simulink model "Sim_model"  (R2024a)
settings: Solver=ode23t  StartTime=0.0  StopTime=7  FixedStep=0.01  MaxStep=0.05  RelTol=1e-3  EnableMultiTasking=on
PreLoadFcn:
  | mdl_puma560
undefined symbols (not defined in the file or in its folder): p560, slcoulomb
libraries: roblocks x3
settings Model: Creator=pic  LastModifiedBy=nicolasaltarelli
settings SolverCC: ZeroCrossControl=DisableAll  AlgebraicLoopSolver=TrustRegion
settings DataIOCC: SaveFormat=Array  SignalLoggingSaveFormat=ModelDataLogs  ReturnWorkspaceOutputs=off  TimeSaveName=t  OutputSaveName=y  ReturnWorkspaceOutputsName=ctorque
settings OptimizationCC: BlockReduction=off  BooleanDataType=off  ExpressionDepthLimit=2147483647  InitFltsAndDblsToZero=on  LifeSpan=inf
settings DebuggingCC: SaveWithParameterizedLinksMsg=none  UnderspecifiedInitializationDetection=Classic  MergeDetectMultiDrivingBlocksExec=none  SignalResolutionControl=TryResolveAllWithWarning  MultiTaskDSMMsg=warning  MultiTaskCondExecSysMsg=none  FcnCallInpInsideContextMsg=warning  UnconnectedInputMsg=warning  UnconnectedOutputMsg=warning  UnconnectedLineMsg=warning  AllowSymbolicDim=off  StateNameClashWarn=warning  SFUnexpectedBacktrackingDiag=warning  SFNoUnconditionalDefaultTransitionDiag=warning  SFExecutionAtInitializationDiag=none  ArithmeticOperatorsInVariantConditions=warning
settings HardwareCC: ProdBitPerPointer=32  ProdBitPerSizeT=32  ProdBitPerPtrDiffT=32  ProdLargestAtomicFloat=None  ProdIntDivRoundTo=Undefined  ProdEndianess=Unspecified  ProdWordSize=32  ProdHWDeviceType=32-bit Generic  TargetUnknown=on
settings ModelReferenceCC: EnableRefExpFcnMdlSchedulingChecks=on  PropagateSignalLabelsOutOfModel=off
settings SFSimCC: SimUseLocalCustomCode=off  CustomCodeUndefinedFunction=UseInterfaceOnly
settings RTWCC: RTWUseLocalCustomCode=off  GPUComputeCapability=3.5
settings CodeAppCC: StateflowObjectComments=on
settings GRTTargetCC: TargetLangStandard=C89/C90 (ANSI)  ModelReferenceCompliant=off  CompOptLevelCompliant=off  CombineOutputUpdateFcns=off  MatFileLogging=off  GRTInterface=on
settings ConfigComp: CovMetricSettings=dw  CovSaveCumulativeToWorkspaceVar=on  CovSaveSingleToWorkspaceVar=on  CovExternalEMLEnable=off

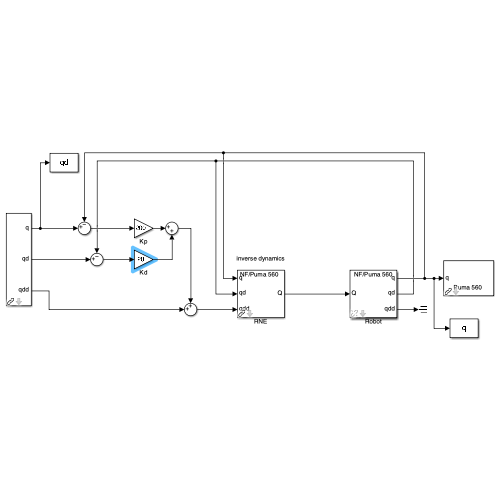
[thumbnail: Simulink's stored preview of the top-level diagram]
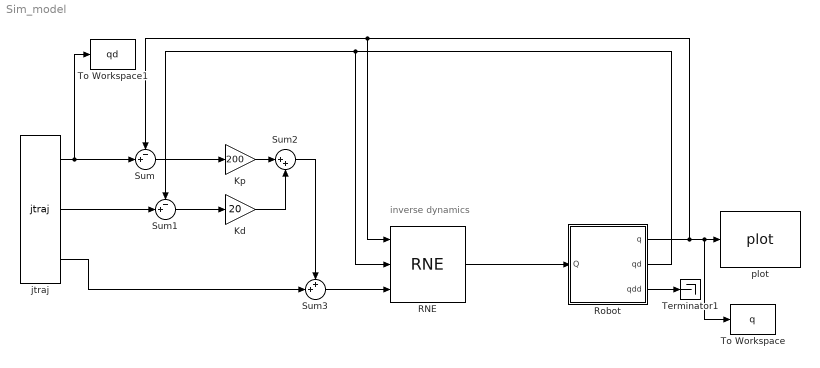
== system Sim_model ==
  note: inverse dynamics
  Kd : Gain  Gain=20  SaturateOnIntegerOverflow=on  OutDataTypeStr=Inherit: Same as input  ParamDataTypeStr=Inherit: Same as input
  Kp : Gain  Gain=200  SaturateOnIntegerOverflow=on  OutDataTypeStr=Inherit: Same as input  ParamDataTypeStr=Inherit: Same as input
  RNE : roblocks/Arm/RNE  robot=p2.nofriction  grav=[0 0 9.81]
  Robot : Subsystem  AncestorBlock=roblocks/Arm/Robot  mask{robot=p560.nofriction, q0=[0 0 0 0 0 0]}
      mask prompts: robot "Robot object"; q0 "Initial state"
      mask help: Rigid-body dynamic model of robot.
      mask init:
      | if isa(robot, 'SerialLink')
      |     rname = robot.name;
      |     %fprintf('**robot name is %s\n', rname);
      | else
      |     rname = '';
      |     n = 0
      | end
      mask Help:
      | Simulates the forward (direct) rigid-body dynamics of the robot described
      | by the given robot object.  For given applied joint torque/force it computes
      | the instaneous joint coordinates, velocities and acclerations.
      | 
      | 
      | <b>Parameters::</b>
      | 
      | robot (SerialLink) a dynamic model of an N-link serial link manipulator
      | q0 (1xN)  Initial joint coordinates
      | 
      | <b>Inputs::</b>
      | 
      | Q (1xN) the generalized joint force (torque or force) required to achieve
      | the motion state (q, qd, qdd).
      | 
      | <b>Outputs::</b>
      | 
      | q (1xN) joint coordinates
      | qd (1xN) joint coordinate velocity
      | qdd (1xN) joint coordinate acceleration
      | 
      | 
      | <b>Notes::</b>
      | 
      | - Required to simulate robot rigid body motion.
      | - Implemented using the recursive Newton-Euler scheme (RNE).
      | - A wrapper for the Toolbox method accel() which in turn depends on the
      |   method rne().
      mask Display:
      | port_label('input', 1, 'Q')
      | port_label('output', 1, 'q')
      | port_label('output', 2, 'qd')
      | port_label('output', 3, 'qdd')
      | text(0.1, 0.9,  rname, 'horizontalAlignment', 'left')
  Sum : Sum  Inputs=-+|  InputSameDT=on  SaturateOnIntegerOverflow=on  OutDataTypeStr=Inherit: Same as first input
  Sum1 : Sum  Inputs=-+|  InputSameDT=on  SaturateOnIntegerOverflow=on  OutDataTypeStr=Inherit: Same as first input
  Sum2 : Sum  Inputs=|++  InputSameDT=on  SaturateOnIntegerOverflow=on  OutDataTypeStr=Inherit: Same as first input
  Sum3 : Sum  Inputs=++|  InputSameDT=on  SaturateOnIntegerOverflow=on  OutDataTypeStr=Inherit: Same as first input
  Terminator1 : Terminator
  To Workspace : ToWorkspace  VariableName=q  SaveFormat=Timeseries  SampleTime=-1
  To Workspace1 : ToWorkspace  VariableName=qd  SaveFormat=Timeseries  SampleTime=-1
  jtraj : roblocks/Toolbox/jtraj  q0=[0 0 0 0 0 0]  qf=[-pi/6 -pi/3 -pi/2 0 0 0]  tmax=5  ts=-1
  plot : roblocks/Arm/plot  robot=p560  fps=10  holdplot=on
  wires:
  Sum/1 -> Kp/1
  Kp/1 -> Sum2/1
  Robot/1(q) -> RNE/1, Sum/1, To Workspace/1, plot/1
  jtraj/1 -> To Workspace1/1, Sum/2
  jtraj/2 -> Sum1/2
  Sum1/1 -> Kd/1
  Kd/1 -> Sum2/2
  Robot/3(qdd) -> Terminator1/1
  Sum3/1 -> RNE/3
  RNE/1 -> Robot/1(Q)
  Robot/2(qd) -> RNE/2, Sum1/1
  jtraj/3 -> Sum3/2
  Sum2/1 -> Sum3/1

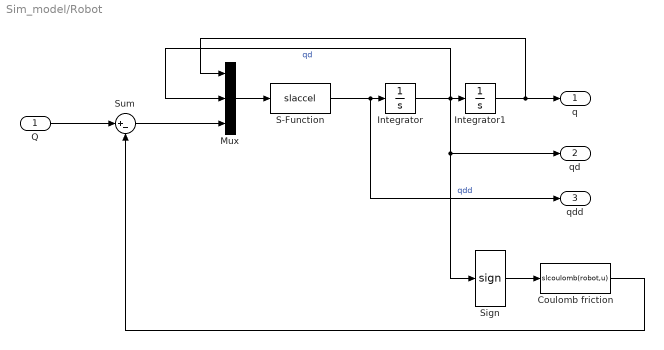
== system Sim_model/Robot ==
  Q : Inport
  Coulomb friction : MATLABFcn  MATLABFcn=slcoulomb(robot,u)  OutputDimensions=[robot.n 1]  Output1D=off
  Integrator : Integrator
  Integrator1 : Integrator  InitialCondition=q0
  Mux : Mux  Inputs=3
  S-Function : S-Function  FunctionName=slaccel  Parameters=robot  SFunctionDeploymentMode=off  EnableBusSupport=off
  Sign : Signum
  Sum : Sum  Inputs=|+-
  q : Outport  VectorParamsAs1DForOutWhenUnconnected=off
  qd : Outport  Port=2  VectorParamsAs1DForOutWhenUnconnected=off
  qdd : Outport  Port=3  VectorParamsAs1DForOutWhenUnconnected=off
  wires:
  S-Function/1 -> qdd/1, Integrator/1  "qdd"
  Mux/1 -> S-Function/1
  Integrator/1 -> Sign/1, qd/1, Integrator1/1, Mux/2  "qd"
  Integrator1/1 -> q/1, Mux/1
  Q/1 -> Sum/1
  Sum/1 -> Mux/3
  Coulomb friction/1 -> Sum/2
  Sign/1 -> Coulomb friction/1
